simulink model "MBD_Prob1"  (R2020a)
settings: Solver=VariableStepAuto  StartTime=0.0  StopTime=10.0  RelTol=1e-3
undefined symbols (not defined in the file): b, K1, K12, M1, M2
settings Model: Creator=Noel Varghese  LastModifiedBy=Noel Varghese

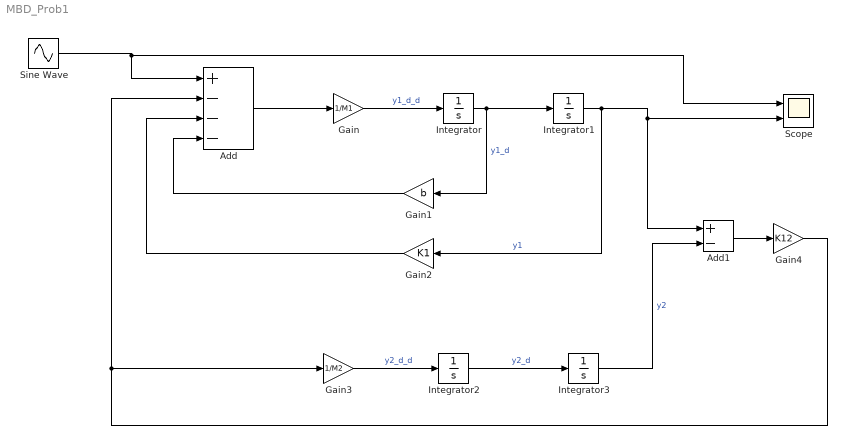
== system MBD_Prob1 ==
  Add : Sum  Inputs=+---
  Add1 : Sum  Inputs=+-
  Gain : Gain  Gain=1/M1
  Gain1 : Gain  Gain=b
  Gain2 : Gain  Gain=K1
  Gain3 : Gain  Gain=1/M2
  Gain4 : Gain  Gain=K12
  Integrator{,1..3} (4 alike) : Integrator
  Scope : Scope  NumInputPorts=2
  Sine Wave : Sin  SampleTime=0
  wires:
  Integrator/1 -> Gain1/1, Integrator1/1  "y1_d"
  Gain/1 -> Integrator/1  "y1_d_d"
  Integrator1/1 -> Gain2/1, Scope/2, Add1/1  "y1"
  Add/1 -> Gain/1
  Gain1/1 -> Add/4
  Gain2/1 -> Add/3
  Integrator2/1 -> Integrator3/1  "y2_d"
  Gain3/1 -> Integrator2/1  "y2_d_d"
  Integrator3/1 -> Add1/2  "y2"
  Add1/1 -> Gain4/1
  Gain4/1 -> Gain3/1, Add/2
  Sine Wave/1 -> Scope/1, Add/1
